simulink library "Arduino_Additional_Lib"  (R2017a)
settings: Solver=VariableStepAuto  StartTime=0.0  StopTime=10.0  RelTol=1e-3
settings Model: Creator=Pavel Roslovets  LastModifiedBy=Pavel Roslovets

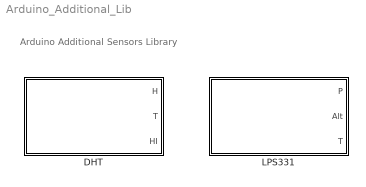
== system Arduino_Additional_Lib ==
  note: Arduino Additional Sensors Library
  DHT : Subsystem  mask(Arduino DHT Sensor){F=off, Pin=8, Tp=11, Ts=0.5}
      mask prompts: F "Output in Fahrenheit (F)"; Pin "Pin number"; Tp "Sensor type"; Ts "Sample Time"
      mask help:
      | Driver based on Adafruit DHT Library
      |
      | Works with DHT11 (11), DHT22 (22), DHT21 (21), AM2301 (21)
      |
      | Output:
      | H - humidity (%)
      | T - Temperature (C or F)
      | HI - HeatIndex (C or F)
      mask Help:
      | <b>Carefully choose Sensor Type parameter:</b>
      | DHT11 - 11
      | DHT22 - 22
      | DHT21 - 21
      | AM2301 - 21
      | 
      | Driver might not work properly with Sample Time is less than 0.3 s
      | 
      | <b>Original Adafruit DHT Library:</b>
      | https://github.com/adafruit/DHT-sensor-library
      mask Display:
      | pic=imread('dht11.png');image(pic,[0.28 0.18 0.45 0.65]);
      | text(0.5, 0.15, 'DHT', 'horizontalAlignment', 'center');
      | color('blue');
      | text(0.55, 0.87, 'ARDUINO', 'horizontalAlignment', 'left');
      | color('black');
  LPS331 : Subsystem  mask(Arduino LPS331 Sensor){Imp=off, Ts=0.1}
      mask prompts: Imp "Umperial units (inHg, ft, F)"; Ts "Sample Time"
      mask help:
      | Driver based on Pololu LPS331 Library
      |
      | Output:
      | P - Pressure (mbar or inHg)
      | A - Altitude (m or ft)
      | T - Temperature (C or F)
      mask Help:
      | LPS331 - I2C barometer
      | 
      | <b>Original Pololu LPS331 Library:</b>
      | https://github.com/pololu/lps331-arduino
      mask Display:
      | pic=imread('lps331.png');image(pic,[0.28 0.18 0.45 0.65]);
      | text(0.5, 0.15, 'LPS331', 'horizontalAlignment', 'center');
      | color('blue');
      | text(0.55, 0.87, 'ARDUINO', 'horizontalAlignment', 'left');
      | color('black');

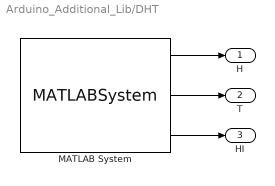
== system Arduino_Additional_Lib/DHT ==
  MATLAB System : MATLABSystem  System=read_dht  Pin=Pin  Sensor=Tp  F=F  SampleTime=Ts
      mask Type: read_dht
      mask Display:
      | disp('read_dht');
      | port_label('output',1,'H');
      | port_label('output',2,'T');
      | port_label('output',3,'HI');
  H : Outport
  T : Outport  Port=2
  HI : Outport  Port=3
  wires:
  MATLAB System/1 -> H/1
  MATLAB System/2 -> T/1
  MATLAB System/3 -> HI/1

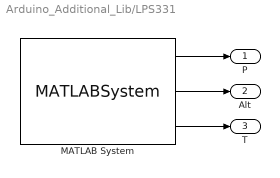
== system Arduino_Additional_Lib/LPS331 ==
  MATLAB System : MATLABSystem  System=read_lps  Imp=Imp  SampleTime=Ts
      mask Type: read_lps
      mask Display:
      | disp('read_lps');
      | port_label('output',1,'P');
      | port_label('output',2,'Alt');
      | port_label('output',3,'T');
  P : Outport
  Alt : Outport  Port=2
  T : Outport  Port=3
  wires:
  MATLAB System/1 -> P/1
  MATLAB System/2 -> Alt/1
  MATLAB System/3 -> T/1
